simulink model "ilcPhase_th"  (R2022a)
settings: Solver=FixedStepAuto  StartTime=0.0  StopTime=10.0  FixedStep=0.001  RelTol=1e-3
libraries: ilcPhase_cl x1
settings Model: Creator=mcobb  LastModifiedBy=lhill8
settings SolverCC: AlgebraicLoopSolver=TrustRegion
settings DebuggingCC: UnconnectedInputMsg=warning  UnconnectedOutputMsg=warning  UnconnectedLineMsg=warning  SFMachineParentedDataDiag=warning  ArithmeticOperatorsInVariantConditions=warning
settings SFSimCC: CustomCodeUndefinedFunction=UseInterfaceOnly

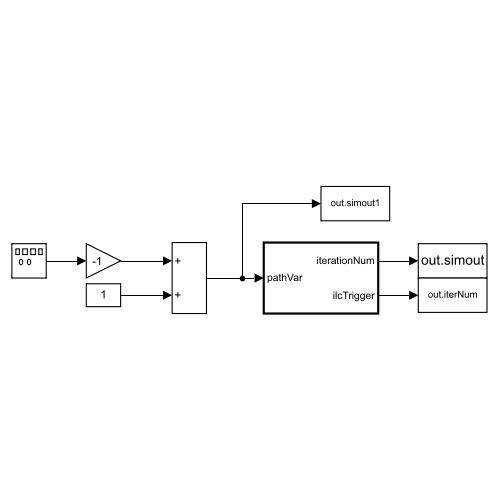
[thumbnail: Simulink's stored preview of the top-level diagram]
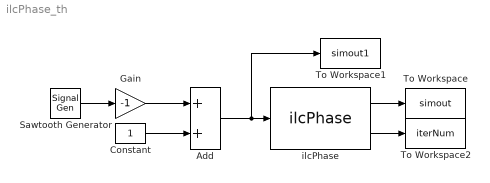
== system ilcPhase_th ==
  Add : Sum
  Constant : Constant
  Gain : Gain  Gain=-1
  Sawtooth Generator : SignalGenerator  WaveForm=sawtooth
  To Workspace : ToWorkspace  VariableName=simout  SaveFormat=Timeseries  SampleTime=-1
  To Workspace1 : ToWorkspace  VariableName=simout1  SaveFormat=Timeseries  SampleTime=-1
  To Workspace2 : ToWorkspace  VariableName=iterNum  SaveFormat=Timeseries  SampleTime=-1
  ilcPhase : ilcPhase_cl/ilcPhase  upperLim=0.1  lowerLim=0.01  numInitLaps=2
  wires:
  ilcPhase/1 -> To Workspace/1
  ilcPhase/2 -> To Workspace2/1
  Constant/1 -> Add/2
  Sawtooth Generator/1 -> Gain/1
  Add/1 -> To Workspace1/1, ilcPhase/1
  Gain/1 -> Add/1
